simulink model "Model_TranslationEngine64"  (R2022b)
settings: Solver=FixedStepDiscrete  StartTime=0.0  StopTime=5  RelTol=1e-3  EnableMultiTasking=on
InitFcn:
  | % Initialize model
  | ModelSettings=BTConfig.GetModelSettings();
  | 
  | ModelSettings.Validate();
  | 
  | ModelInit;
  | 
  | 
  | % load library data
  | GainLibrary_data;
  | % Load saved values from partition process
  | CapturedConstMask.LoadMapFromFile(bdroot)
StartFcn:
  | % make sure all the simulated RTC requests are found
  | %RTC_SIM_OBJ.ValidateREQs();
undefined symbols (not defined in the file or in its folder): AA, BPLP, Column, NumHFRefBPF, NumHFRefLPF, NumMusicChannels, Row, VolumeMuteConfig
libraries: TuneVar x925, TOP x490, FeaturePath x111, CapturedConstLib x52
(part 24 of 34)

== system Model_TranslationEngine64/ModelPreAmp/DecRate/Medusa5H1/SleepingBeauty/SleepingBeauty/Enabled/SleepingBeautyDR/InnerLink ==
  Captured Tune Const : CapturedConstLib/CapturedConst  TriggerInit=[155 22 255 58]  Role=Automatic
      settings: SourceProductName=Bose Talaria
  FeaturePath : FeaturePath/FeaturePath  FeatureName=SleepingBeautyDR  IsGroup=off  GroupNumber=-1  IsModule=off  TriggerInit=[-415 -561 -300 -454]
      settings: SourceProductName=Bose Talaria
  TOP : TOP/TOP  TriggerInit=[555 -30 785 30]  TopName=ChannelToRamperMap  DataTypeOut=single  BankNumber=0  PreOverlay=false  PostOverlay=false  Role=Automatic
      settings: SourceProductName=Bose Talaria
  TranslateTrigger : TuneVar/TranslateTrigger  TriggerInit=[421 -160 459 -105]
      settings: SourceProductName=Bose Talaria
  TuneTOP : Subsystem  Description=Defines the index at which the index is at the center, i.e. neither towards the left nor the right sides.  mask(Talaria Trivial Tune TOP){TriggerInit=[-595 -93 -425 -37], TopName=Offset, TuneName=Offset, DataTypeOut=single, MaskValue=Config.DefaultOffset, TunabilityNumber=1, MinValue=[], MaxValue=[], BankNumber=0, PreOverlay=false, PostOverlay=false, UseSameName=on}
      mask prompts: TriggerInit "Hidden: MoveFcn redraw"; TopName "Name:"; TuneName "Name of TuneVar:"; DataTypeOut "Data type:"; MaskValue "Default Value:"; TunabilityNumber "Tunability:"; MinValue "Min Value:"; MaxValue "Max Value:"; BankNumber "Target memory bank number:"; PreOverlay "Requires pre-overlay action:"; PostOverlay "Requires post-overlay action:"; UseSameName "Use same name for tune variable and TOP"
      mask help: The TuneTOP block encapsultes a Target Overlay Parameter, a Tune Variable, and a Trivial Translation between them.
      mask init:
      | [ok,activeTopPath,activeTunePath] = TuneTOP_Mask.Init(gcbh);
      settings: MoveFcn=TuneTOP_Mask.CB_TriggerInit(gcbh);
      mask Callback TriggerInit: TuneTOP_Mask.CB_TriggerInit(gcbh);
      mask TypeOptions TopName: TOP/TopName
      mask TypeOptions TuneName: Tune Variable/TuneName
      mask TypeOptions DataTypeOut: TOP/DataTypeOut
      mask TypeOptions MaskValue: Tune Variable/MaskValue
      mask TypeOptions TunabilityNumber: Tune Variable/TunabilityNumber
      mask Callback TunabilityNumber: TuneVarMask.CB_TunabilityNumber(gcbh);
      mask TypeOptions MinValue: Tune Variable/MinValue
      mask TypeOptions MaxValue: Tune Variable/MaxValue
      mask TypeOptions BankNumber: TOP/BankNumber
      mask TypeOptions PreOverlay: TOP/PreOverlay
      mask TypeOptions PostOverlay: TOP/PostOverlay
      mask Callback UseSameName: TuneTOP_Mask.CB_UseSameName(gcbh);
      mask DialogControl toolPanel Prompt: Tuning Tool Hints
      mask DialogControl DescriptionGroup Prompt: Description
      mask DialogControl EditDescription Prompt: Edit Description
      mask DialogControl EditDescription Callback: TuneTOP_Mask.CB_EditDescription(gcbh);
      mask DialogControl TunabilityText Prompt: Easy: Changes nearly every tuning.
      mask DialogControl AdvancedPanel Prompt: Advanced
      mask DialogControl ConvertToFullTranslation Prompt: Irreversible conversion to full translation
      mask DialogControl ConvertToFullTranslation Callback: TuneTOP_Mask.CB_ConvertToFullTranslation(gcbh);
      mask DialogControl ErrorContainer Prompt: Error Messages
      mask Display:
      | % retrieve icon definition
      | [path,w,h] = TuneTOP_Mask.Icon();
      | 
      | % retrieve the block's pixel size
      | pos = get(gcbh,'position');
      | bw = pos(3) - pos(1);
      | bh = pos(4) - pos(2);
      | 
      | % draw centered icon
      | xAdj = bw/2 - w/2 + 5;
      | yAdj = bh/2 - h/2 + 4;
      | for i=1:length(path)
      | 	patch(path(i).x+xAdj, path(i).y+yAdj, path(i).rgb);
      | end
      | 
      | % show the top name or an X
      | if (exist('ok','var') && ok)
      | 	text(bw*0.5, bh*0.2, activeTopPath, 'horizontalAlignment', 'center');
      | 	patch(0,0,[1 1 1]);
      | 	patch(bw,bh,[1 1 1]);
      | else
      | 	tx=bw*0.03;
      | 	ty=bh*0.03;
      | 	patch([0 tx bw bw-tx], [ty 0 bh-ty bh], [1 0 0]);
      | 	patch([0 bw-tx bw tx], [bh-ty 0 ty bh], [1 0 0]);
      | end
  TuneTOP1 : Subsystem  mask(Talaria Trivial Tune TOP){TriggerInit=[135 -393 305 -337], TopName=RampTime, TuneName=RampTime, DataTypeOut=single, MaskValue=30, TunabilityNumber=1, MinValue=[], MaxValue=[], BankNumber=0, PreOverlay=false, PostOverlay=false, UseSameName=on}
      mask prompts: TriggerInit "Hidden: MoveFcn redraw"; TopName "Name:"; TuneName "Name of TuneVar:"; DataTypeOut "Data type:"; MaskValue "Default Value:"; TunabilityNumber "Tunability:"; MinValue "Min Value:"; MaxValue "Max Value:"; BankNumber "Target memory bank number:"; PreOverlay "Requires pre-overlay action:"; PostOverlay "Requires post-overlay action:"; UseSameName "Use same name for tune variable and TOP"
      mask help: The TuneTOP block encapsultes a Target Overlay Parameter, a Tune Variable, and a Trivial Translation between them.
      mask init:
      | [ok,activeTopPath,activeTunePath] = TuneTOP_Mask.Init(gcbh);
      settings: MoveFcn=TuneTOP_Mask.CB_TriggerInit(gcbh);
      mask Callback TriggerInit: TuneTOP_Mask.CB_TriggerInit(gcbh);
      mask TypeOptions TopName: TOP/TopName
      mask TypeOptions TuneName: Tune Variable/TuneName
      mask TypeOptions DataTypeOut: TOP/DataTypeOut
      mask TypeOptions MaskValue: Tune Variable/MaskValue
      mask TypeOptions TunabilityNumber: Tune Variable/TunabilityNumber
      mask Callback TunabilityNumber: TuneVarMask.CB_TunabilityNumber(gcbh);
      mask TypeOptions MinValue: Tune Variable/MinValue
      mask TypeOptions MaxValue: Tune Variable/MaxValue
      mask TypeOptions BankNumber: TOP/BankNumber
      mask TypeOptions PreOverlay: TOP/PreOverlay
      mask TypeOptions PostOverlay: TOP/PostOverlay
      mask Callback UseSameName: TuneTOP_Mask.CB_UseSameName(gcbh);
      mask DialogControl toolPanel Prompt: Tuning Tool Hints
      mask DialogControl DescriptionGroup Prompt: Description
      mask DialogControl EditDescription Prompt: Edit Description
      mask DialogControl EditDescription Callback: TuneTOP_Mask.CB_EditDescription(gcbh);
      mask DialogControl TunabilityText Prompt: Easy: Changes nearly every tuning.
      mask DialogControl AdvancedPanel Prompt: Advanced
      mask DialogControl ConvertToFullTranslation Prompt: Irreversible conversion to full translation
      mask DialogControl ConvertToFullTranslation Callback: TuneTOP_Mask.CB_ConvertToFullTranslation(gcbh);
      mask DialogControl ErrorContainer Prompt: Error Messages
      mask Display:
      | % retrieve icon definition
      | [path,w,h] = TuneTOP_Mask.Icon();
      | 
      | % retrieve the block's pixel size
      | pos = get(gcbh,'position');
      | bw = pos(3) - pos(1);
      | bh = pos(4) - pos(2);
      | 
      | % draw centered icon
      | xAdj = bw/2 - w/2 + 5;
      | yAdj = bh/2 - h/2 + 4;
      | for i=1:length(path)
      | 	patch(path(i).x+xAdj, path(i).y+yAdj, path(i).rgb);
      | end
      | 
      | % show the top name or an X
      | if (exist('ok','var') && ok)
      | 	text(bw*0.5, bh*0.2, activeTopPath, 'horizontalAlignment', 'center');
      | 	patch(0,0,[1 1 1]);
      | 	patch(bw,bh,[1 1 1]);
      | else
      | 	tx=bw*0.03;
      | 	ty=bh*0.03;
      | 	patch([0 tx bw bw-tx], [ty 0 bh-ty bh], [1 0 0]);
      | 	patch([0 bw-tx bw tx], [bh-ty 0 ty bh], [1 0 0]);
      | end
  TuneTOP2 : Subsystem  Description=Defines the index at which the index is at the center, i.e. neither towards the left nor the right sides.  mask(Talaria Trivial Tune TOP){TriggerInit=[-595 17 -425 73], TopName=MutesBass, TuneName=MutesBass, DataTypeOut=single, MaskValue=Config.DefaultSilentExtremeMutesBass, TunabilityNumber=1, MinValue=[], MaxValue=[], BankNumber=0, PreOverlay=false, PostOverlay=false, UseSameName=on}
      mask prompts: TriggerInit "Hidden: MoveFcn redraw"; TopName "Name:"; TuneName "Name of TuneVar:"; DataTypeOut "Data type:"; MaskValue "Default Value:"; TunabilityNumber "Tunability:"; MinValue "Min Value:"; MaxValue "Max Value:"; BankNumber "Target memory bank number:"; PreOverlay "Requires pre-overlay action:"; PostOverlay "Requires post-overlay action:"; UseSameName "Use same name for tune variable and TOP"
      mask help: The TuneTOP block encapsultes a Target Overlay Parameter, a Tune Variable, and a Trivial Translation between them.
      mask init:
      | [ok,activeTopPath,activeTunePath] = TuneTOP_Mask.Init(gcbh);
      settings: MoveFcn=TuneTOP_Mask.CB_TriggerInit(gcbh);
      mask Callback TriggerInit: TuneTOP_Mask.CB_TriggerInit(gcbh);
      mask TypeOptions TopName: TOP/TopName
      mask TypeOptions TuneName: Tune Variable/TuneName
      mask TypeOptions DataTypeOut: TOP/DataTypeOut
      mask TypeOptions MaskValue: Tune Variable/MaskValue
      mask TypeOptions TunabilityNumber: Tune Variable/TunabilityNumber
      mask Callback TunabilityNumber: TuneVarMask.CB_TunabilityNumber(gcbh);
      mask TypeOptions MinValue: Tune Variable/MinValue
      mask TypeOptions MaxValue: Tune Variable/MaxValue
      mask TypeOptions BankNumber: TOP/BankNumber
      mask TypeOptions PreOverlay: TOP/PreOverlay
      mask TypeOptions PostOverlay: TOP/PostOverlay
      mask Callback UseSameName: TuneTOP_Mask.CB_UseSameName(gcbh);
      mask DialogControl toolPanel Prompt: Tuning Tool Hints
      mask DialogControl DescriptionGroup Prompt: Description
      mask DialogControl EditDescription Prompt: Edit Description
      mask DialogControl EditDescription Callback: TuneTOP_Mask.CB_EditDescription(gcbh);
      mask DialogControl TunabilityText Prompt: Easy: Changes nearly every tuning.
      mask DialogControl AdvancedPanel Prompt: Advanced
      mask DialogControl ConvertToFullTranslation Prompt: Irreversible conversion to full translation
      mask DialogControl ConvertToFullTranslation Callback: TuneTOP_Mask.CB_ConvertToFullTranslation(gcbh);
      mask DialogControl ErrorContainer Prompt: Error Messages
      mask Display:
      | % retrieve icon definition
      | [path,w,h] = TuneTOP_Mask.Icon();
      | 
      | % retrieve the block's pixel size
      | pos = get(gcbh,'position');
      | bw = pos(3) - pos(1);
      | bh = pos(4) - pos(2);
      | 
      | % draw centered icon
      | xAdj = bw/2 - w/2 + 5;
      | yAdj = bh/2 - h/2 + 4;
      | for i=1:length(path)
      | 	patch(path(i).x+xAdj, path(i).y+yAdj, path(i).rgb);
      | end
      | 
      | % show the top name or an X
      | if (exist('ok','var') && ok)
      | 	text(bw*0.5, bh*0.2, activeTopPath, 'horizontalAlignment', 'center');
      | 	patch(0,0,[1 1 1]);
      | 	patch(bw,bh,[1 1 1]);
      | else
      | 	tx=bw*0.03;
      | 	ty=bh*0.03;
      | 	patch([0 tx bw bw-tx], [ty 0 bh-ty bh], [1 0 0]);
      | 	patch([0 bw-tx bw tx], [bh-ty 0 ty bh], [1 0 0]);
      | end
  TuneVarChannelRamperMap : TuneVar/TuneVar  TuneName=ChannelToRamperMap  SpecifyMaxSize=off  VariableDim=1 (Row)  MaxSize=[1 1]  TunabilityNumber=1  MinValue=[]  MaxValue=[]  TriggerInit=[70 -65 280 -15]  MaskValue=Config.ChanToRampMap
      settings: SourceProductName=Bose Talaria
  TuneVarTable : Subsystem
  channel_ramper_translation : MATLAB Function  TreatAsAtomicUnit=on  mask{MaskNumRampers=Config.NumRampers}
  wires:
  TranslateTrigger/1 -> channel_ramper_translation/Trigger
  TuneVarChannelRamperMap/1 -> channel_ramper_translation/1(TuneChanRampMap)  "ChannelToRamperMap"
  channel_ramper_translation/1(ChanRampMap) -> TOP/1
  Captured Tune Const/1 -> channel_ramper_translation/2(channelCount)

== system Model_TranslationEngine64/ModelPreAmp/DecRate/Medusa5H1/SleepingBeauty/SleepingBeauty/Enabled/SleepingBeautyFR/InnerLink ==
  Captured Tune Const : CapturedConstLib/CapturedConst  TriggerInit=[155 22 255 58]  Role=Automatic
      settings: SourceProductName=Bose Talaria
  FeaturePath : FeaturePath/FeaturePath  FeatureName=SleepingBeautyFR  IsGroup=off  GroupNumber=-1  IsModule=off  TriggerInit=[-415 -561 -300 -454]
      settings: SourceProductName=Bose Talaria
  TOP : TOP/TOP  TriggerInit=[555 -30 785 30]  TopName=ChannelToRamperMap  DataTypeOut=single  BankNumber=0  PreOverlay=false  PostOverlay=false  Role=Automatic
      settings: SourceProductName=Bose Talaria
  TranslateTrigger : TuneVar/TranslateTrigger  TriggerInit=[421 -160 459 -105]
      settings: SourceProductName=Bose Talaria
  TuneTOP : Subsystem  Description=Defines the index at which the index is at the center, i.e. neither towards the left nor the right sides.  mask(Talaria Trivial Tune TOP){TriggerInit=[-595 -93 -425 -37], TopName=Offset, TuneName=Offset, DataTypeOut=single, MaskValue=Config.DefaultOffset, TunabilityNumber=1, MinValue=[], MaxValue=[], BankNumber=0, PreOverlay=false, PostOverlay=false, UseSameName=on}
      mask prompts: TriggerInit "Hidden: MoveFcn redraw"; TopName "Name:"; TuneName "Name of TuneVar:"; DataTypeOut "Data type:"; MaskValue "Default Value:"; TunabilityNumber "Tunability:"; MinValue "Min Value:"; MaxValue "Max Value:"; BankNumber "Target memory bank number:"; PreOverlay "Requires pre-overlay action:"; PostOverlay "Requires post-overlay action:"; UseSameName "Use same name for tune variable and TOP"
      mask help: The TuneTOP block encapsultes a Target Overlay Parameter, a Tune Variable, and a Trivial Translation between them.
      mask init:
      | [ok,activeTopPath,activeTunePath] = TuneTOP_Mask.Init(gcbh);
      settings: MoveFcn=TuneTOP_Mask.CB_TriggerInit(gcbh);
      mask Callback TriggerInit: TuneTOP_Mask.CB_TriggerInit(gcbh);
      mask TypeOptions TopName: TOP/TopName
      mask TypeOptions TuneName: Tune Variable/TuneName
      mask TypeOptions DataTypeOut: TOP/DataTypeOut
      mask TypeOptions MaskValue: Tune Variable/MaskValue
      mask TypeOptions TunabilityNumber: Tune Variable/TunabilityNumber
      mask Callback TunabilityNumber: TuneVarMask.CB_TunabilityNumber(gcbh);
      mask TypeOptions MinValue: Tune Variable/MinValue
      mask TypeOptions MaxValue: Tune Variable/MaxValue
      mask TypeOptions BankNumber: TOP/BankNumber
      mask TypeOptions PreOverlay: TOP/PreOverlay
      mask TypeOptions PostOverlay: TOP/PostOverlay
      mask Callback UseSameName: TuneTOP_Mask.CB_UseSameName(gcbh);
      mask DialogControl toolPanel Prompt: Tuning Tool Hints
      mask DialogControl DescriptionGroup Prompt: Description
      mask DialogControl EditDescription Prompt: Edit Description
      mask DialogControl EditDescription Callback: TuneTOP_Mask.CB_EditDescription(gcbh);
      mask DialogControl TunabilityText Prompt: Easy: Changes nearly every tuning.
      mask DialogControl AdvancedPanel Prompt: Advanced
      mask DialogControl ConvertToFullTranslation Prompt: Irreversible conversion to full translation
      mask DialogControl ConvertToFullTranslation Callback: TuneTOP_Mask.CB_ConvertToFullTranslation(gcbh);
      mask DialogControl ErrorContainer Prompt: Error Messages
      mask Display:
      | % retrieve icon definition
      | [path,w,h] = TuneTOP_Mask.Icon();
      | 
      | % retrieve the block's pixel size
      | pos = get(gcbh,'position');
      | bw = pos(3) - pos(1);
      | bh = pos(4) - pos(2);
      | 
      | % draw centered icon
      | xAdj = bw/2 - w/2 + 5;
      | yAdj = bh/2 - h/2 + 4;
      | for i=1:length(path)
      | 	patch(path(i).x+xAdj, path(i).y+yAdj, path(i).rgb);
      | end
      | 
      | % show the top name or an X
      | if (exist('ok','var') && ok)
      | 	text(bw*0.5, bh*0.2, activeTopPath, 'horizontalAlignment', 'center');
      | 	patch(0,0,[1 1 1]);
      | 	patch(bw,bh,[1 1 1]);
      | else
      | 	tx=bw*0.03;
      | 	ty=bh*0.03;
      | 	patch([0 tx bw bw-tx], [ty 0 bh-ty bh], [1 0 0]);
      | 	patch([0 bw-tx bw tx], [bh-ty 0 ty bh], [1 0 0]);
      | end
  TuneTOP1 : Subsystem  mask(Talaria Trivial Tune TOP){TriggerInit=[135 -393 305 -337], TopName=RampTime, TuneName=RampTime, DataTypeOut=single, MaskValue=30, TunabilityNumber=1, MinValue=[], MaxValue=[], BankNumber=0, PreOverlay=false, PostOverlay=false, UseSameName=on}
      mask prompts: TriggerInit "Hidden: MoveFcn redraw"; TopName "Name:"; TuneName "Name of TuneVar:"; DataTypeOut "Data type:"; MaskValue "Default Value:"; TunabilityNumber "Tunability:"; MinValue "Min Value:"; MaxValue "Max Value:"; BankNumber "Target memory bank number:"; PreOverlay "Requires pre-overlay action:"; PostOverlay "Requires post-overlay action:"; UseSameName "Use same name for tune variable and TOP"
      mask help: The TuneTOP block encapsultes a Target Overlay Parameter, a Tune Variable, and a Trivial Translation between them.
      mask init:
      | [ok,activeTopPath,activeTunePath] = TuneTOP_Mask.Init(gcbh);
      settings: MoveFcn=TuneTOP_Mask.CB_TriggerInit(gcbh);
      mask Callback TriggerInit: TuneTOP_Mask.CB_TriggerInit(gcbh);
      mask TypeOptions TopName: TOP/TopName
      mask TypeOptions TuneName: Tune Variable/TuneName
      mask TypeOptions DataTypeOut: TOP/DataTypeOut
      mask TypeOptions MaskValue: Tune Variable/MaskValue
      mask TypeOptions TunabilityNumber: Tune Variable/TunabilityNumber
      mask Callback TunabilityNumber: TuneVarMask.CB_TunabilityNumber(gcbh);
      mask TypeOptions MinValue: Tune Variable/MinValue
      mask TypeOptions MaxValue: Tune Variable/MaxValue
      mask TypeOptions BankNumber: TOP/BankNumber
      mask TypeOptions PreOverlay: TOP/PreOverlay
      mask TypeOptions PostOverlay: TOP/PostOverlay
      mask Callback UseSameName: TuneTOP_Mask.CB_UseSameName(gcbh);
      mask DialogControl toolPanel Prompt: Tuning Tool Hints
      mask DialogControl DescriptionGroup Prompt: Description
      mask DialogControl EditDescription Prompt: Edit Description
      mask DialogControl EditDescription Callback: TuneTOP_Mask.CB_EditDescription(gcbh);
      mask DialogControl TunabilityText Prompt: Easy: Changes nearly every tuning.
      mask DialogControl AdvancedPanel Prompt: Advanced
      mask DialogControl ConvertToFullTranslation Prompt: Irreversible conversion to full translation
      mask DialogControl ConvertToFullTranslation Callback: TuneTOP_Mask.CB_ConvertToFullTranslation(gcbh);
      mask DialogControl ErrorContainer Prompt: Error Messages
      mask Display:
      | % retrieve icon definition
      | [path,w,h] = TuneTOP_Mask.Icon();
      | 
      | % retrieve the block's pixel size
      | pos = get(gcbh,'position');
      | bw = pos(3) - pos(1);
      | bh = pos(4) - pos(2);
      | 
      | % draw centered icon
      | xAdj = bw/2 - w/2 + 5;
      | yAdj = bh/2 - h/2 + 4;
      | for i=1:length(path)
      | 	patch(path(i).x+xAdj, path(i).y+yAdj, path(i).rgb);
      | end
      | 
      | % show the top name or an X
      | if (exist('ok','var') && ok)
      | 	text(bw*0.5, bh*0.2, activeTopPath, 'horizontalAlignment', 'center');
      | 	patch(0,0,[1 1 1]);
      | 	patch(bw,bh,[1 1 1]);
      | else
      | 	tx=bw*0.03;
      | 	ty=bh*0.03;
      | 	patch([0 tx bw bw-tx], [ty 0 bh-ty bh], [1 0 0]);
      | 	patch([0 bw-tx bw tx], [bh-ty 0 ty bh], [1 0 0]);
      | end
  TuneTOP2 : Subsystem  Description=Defines the index at which the index is at the center, i.e. neither towards the left nor the right sides.  mask(Talaria Trivial Tune TOP){TriggerInit=[-595 17 -425 73], TopName=MutesBass, TuneName=MutesBass, DataTypeOut=single, MaskValue=Config.DefaultSilentExtremeMutesBass, TunabilityNumber=1, MinValue=[], MaxValue=[], BankNumber=0, PreOverlay=false, PostOverlay=false, UseSameName=on}
      mask prompts: TriggerInit "Hidden: MoveFcn redraw"; TopName "Name:"; TuneName "Name of TuneVar:"; DataTypeOut "Data type:"; MaskValue "Default Value:"; TunabilityNumber "Tunability:"; MinValue "Min Value:"; MaxValue "Max Value:"; BankNumber "Target memory bank number:"; PreOverlay "Requires pre-overlay action:"; PostOverlay "Requires post-overlay action:"; UseSameName "Use same name for tune variable and TOP"
      mask help: The TuneTOP block encapsultes a Target Overlay Parameter, a Tune Variable, and a Trivial Translation between them.
      mask init:
      | [ok,activeTopPath,activeTunePath] = TuneTOP_Mask.Init(gcbh);
      settings: MoveFcn=TuneTOP_Mask.CB_TriggerInit(gcbh);
      mask Callback TriggerInit: TuneTOP_Mask.CB_TriggerInit(gcbh);
      mask TypeOptions TopName: TOP/TopName
      mask TypeOptions TuneName: Tune Variable/TuneName
      mask TypeOptions DataTypeOut: TOP/DataTypeOut
      mask TypeOptions MaskValue: Tune Variable/MaskValue
      mask TypeOptions TunabilityNumber: Tune Variable/TunabilityNumber
      mask Callback TunabilityNumber: TuneVarMask.CB_TunabilityNumber(gcbh);
      mask TypeOptions MinValue: Tune Variable/MinValue
      mask TypeOptions MaxValue: Tune Variable/MaxValue
      mask TypeOptions BankNumber: TOP/BankNumber
      mask TypeOptions PreOverlay: TOP/PreOverlay
      mask TypeOptions PostOverlay: TOP/PostOverlay
      mask Callback UseSameName: TuneTOP_Mask.CB_UseSameName(gcbh);
      mask DialogControl toolPanel Prompt: Tuning Tool Hints
      mask DialogControl DescriptionGroup Prompt: Description
      mask DialogControl EditDescription Prompt: Edit Description
      mask DialogControl EditDescription Callback: TuneTOP_Mask.CB_EditDescription(gcbh);
      mask DialogControl TunabilityText Prompt: Easy: Changes nearly every tuning.
      mask DialogControl AdvancedPanel Prompt: Advanced
      mask DialogControl ConvertToFullTranslation Prompt: Irreversible conversion to full translation
      mask DialogControl ConvertToFullTranslation Callback: TuneTOP_Mask.CB_ConvertToFullTranslation(gcbh);
      mask DialogControl ErrorContainer Prompt: Error Messages
      mask Display:
      | % retrieve icon definition
      | [path,w,h] = TuneTOP_Mask.Icon();
      | 
      | % retrieve the block's pixel size
      | pos = get(gcbh,'position');
      | bw = pos(3) - pos(1);
      | bh = pos(4) - pos(2);
      | 
      | % draw centered icon
      | xAdj = bw/2 - w/2 + 5;
      | yAdj = bh/2 - h/2 + 4;
      | for i=1:length(path)
      | 	patch(path(i).x+xAdj, path(i).y+yAdj, path(i).rgb);
      | end
      | 
      | % show the top name or an X
      | if (exist('ok','var') && ok)
      | 	text(bw*0.5, bh*0.2, activeTopPath, 'horizontalAlignment', 'center');
      | 	patch(0,0,[1 1 1]);
      | 	patch(bw,bh,[1 1 1]);
      | else
      | 	tx=bw*0.03;
      | 	ty=bh*0.03;
      | 	patch([0 tx bw bw-tx], [ty 0 bh-ty bh], [1 0 0]);
      | 	patch([0 bw-tx bw tx], [bh-ty 0 ty bh], [1 0 0]);
      | end
  TuneVarChannelRamperMap : TuneVar/TuneVar  TuneName=ChannelToRamperMap  SpecifyMaxSize=off  VariableDim=1 (Row)  MaxSize=[1 1]  TunabilityNumber=1  MinValue=[]  MaxValue=[]  TriggerInit=[70 -65 280 -15]  MaskValue=Config.ChanToRampMap
      settings: SourceProductName=Bose Talaria
  TuneVarTable : Subsystem
  channel_ramper_translation : MATLAB Function  TreatAsAtomicUnit=on  mask{MaskNumRampers=Config.NumRampers}
  wires:
  TranslateTrigger/1 -> channel_ramper_translation/Trigger
  TuneVarChannelRamperMap/1 -> channel_ramper_translation/1(TuneChanRampMap)  "ChannelToRamperMap"
  channel_ramper_translation/1(ChanRampMap) -> TOP/1
  Captured Tune Const/1 -> channel_ramper_translation/2(channelCount)

== system Model_TranslationEngine64/ModelPreAmp/DecRate/Medusa5H1/VLS/Crosstalk Cancellation/Pooliir with Non-Trivial Translations/InnerLink/PoolIirTunableWithReset ==
  CapturedTuneConst : CapturedConstLib/CapturedConst  TriggerInit=[-600 302 -500 338]  Role=Automatic
      settings: SourceProductName=Bose Talaria
  FeaturePath : FeaturePath/FeaturePath  FeatureName=IIR  IsGroup=off  GroupNumber=-1  IsModule=off  TriggerInit=[-750 -81 -635 26]
      settings: SourceProductName=Bose Talaria
  TOP : TOP/TOP  TriggerInit=[-145 187 5 243]  TopName=PooliirNumStages  DataTypeOut=uint32  BankNumber=0  PreOverlay=false  PostOverlay=Config.VariantObj.PostOverlayRequired  Role=Automatic
      settings: SourceProductName=Bose Talaria
  TOP1 : TOP/TOP  TriggerInit=[-140 277 10 333]  TopName=pooliirCoeffs  DataTypeOut=single  BankNumber=0  PreOverlay=false  PostOverlay=Config.VariantObj.PostOverlayRequired  Role=Automatic
      settings: SourceProductName=Bose Talaria
  TranslateTrigger : TuneVar/TranslateTrigger  TriggerInit=[-339 35 -301 90]
      settings: SourceProductName=Bose Talaria
  Translation : MATLAB Function  TreatAsAtomicUnit=on  mask{MaxNumStages=Config.MaxNumStages, VariantUint8=Config.Variant.Uint8Str}
      mask prompts: VariantUint8 "Variant"
  Tune Variable1 : TuneVar/TuneVar  TuneName=numStages  SpecifyMaxSize=off  VariableDim=1 (Row)  MaxSize=[1 1]  TunabilityNumber=1  MinValue=[]  MaxValue=[]  TriggerInit=[-750 235 -580 285]  MaskValue=Config.TuneDefaults.NumStages
      settings: SourceProductName=Bose Talaria
  Tune Variable2 : TuneVar/TuneVar  TuneName=sosCoefficients  SpecifyMaxSize=on  VariableDim=1 (Row)  MaxSize=[Config.MaxNumStages 6]  TunabilityNumber=1  MinValue=[]  MaxValue=[]  TriggerInit=[-750 175 -580 225]  MaskValue=Config.TuneDefaults.SosCoefficients
      settings: SourceProductName=Bose Talaria
  wires:
  CapturedTuneConst/1 -> Translation/3(NumChannels)
  Tune Variable1/1 -> Translation/2(NumStages)  "numStages"
  Translation/1(PoolNumStages) -> TOP/1
  Translation/2(PoolCoeffs) -> TOP1/1
  Tune Variable2/1 -> Translation/1(RawSOS)  "sosCoefficients"
  TranslateTrigger/1 -> Translation/Trigger

== system Model_TranslationEngine64/ModelPreAmp/PreAmpPart1/NEARPreAmp/Monoizer/Monoizer/MonoizerStereo/MonoizerCalc/TuneTOP1 ==
  TOP : TOP/TOP  TriggerInit=[440 20 585 80]  TopName=G  DataTypeOut=single  BankNumber=BankNumber  PreOverlay=PreOverlay  PostOverlay=PostOverlay  Role=Automatic
      settings: SourceProductName=Bose Talaria
  TrivialTranslation : TuneVar/TrivialTranslation  TriggerInit=[300 28 350 72]
      settings: SourceProductName=Bose Talaria
  Tune Variable : TuneVar/TuneVar  TuneName=G  SpecifyMaxSize=off  VariableDim=1 (Row)  MaxSize=[1 1]  TunabilityNumber=1  MinValue=MinValue  MaxValue=MaxValue  TriggerInit=[20 25 190 75]  MaskValue=MaskValue
      settings: SourceProductName=Bose Talaria
  wires:
  Tune Variable/1 -> TrivialTranslation/1  "G"
  TrivialTranslation/1 -> TOP/1

== system Model_TranslationEngine64/ModelPreAmp/DecRate/AudioPilot35/Audiopilot_3_5/NoiseEstimationVariant/RegularNoiseEstimation/HFNoiseEstimatorCoh/HfNoiseMusicSeparation /RefPowerMin ==
  RefPowerMin : TOP/TOP  TriggerInit=[440 20 585 80]  TopName=RefPowerMin  DataTypeOut=single  BankNumber=0  PreOverlay=false  PostOverlay=false  Role=Automatic
      settings: SourceProductName=Bose Talaria
  TranslateTrigger : TuneVar/TranslateTrigger  TriggerInit=[306 -100 344 -45]
      settings: SourceProductName=Bose Talaria
  Tune Variable : TuneVar/TuneVar  TuneName=RefPowerMinDb  SpecifyMaxSize=off  VariableDim=1 (Row)  MaxSize=[1 1]  TunabilityNumber=1  MinValue=[]  MaxValue=[]  TriggerInit=[-25 25 145 75]  MaskValue=Config.RefPowerMinDb
      settings: SourceProductName=Bose Talaria
  undB : MATLAB Function  TreatAsAtomicUnit=on
  wires:
  Tune Variable/1 -> undB/1(Tune)  "RefPowerMinDb"
  undB/1(TOP) -> RefPowerMin/1
  TranslateTrigger/1 -> undB/Trigger

== system Model_TranslationEngine64/ModelPreAmp/DecRate/AudioPilot35/Audiopilot_3_5/NoiseEstimationVariant/RegularNoiseEstimation/HFNoiseEstimatorCoh/PostProcessing/HfImpulseRejection ==
  note: Impulse and Speech Rejection
  ComputeSmoothingFactor : Subsystem
  FeaturePath : FeaturePath/FeaturePath  FeatureName=ImpulseRejection  IsGroup=off  GroupNumber=-1  IsModule=off  TriggerInit=[750 304 1100 406]
      settings: SourceProductName=Bose Talaria
  "IntermediateCalculation1 " : Subsystem
  MinSearch : Subsystem
  SmoothingNoiseFloor : Subsystem

== system Model_TranslationEngine64/ModelPreAmp/DecRate/AudioPilot35/Audiopilot_3_5/NoiseEstimationVariant/RegularNoiseEstimation/HFNoiseEstimatorCoh/PostProcessing/HfSlew ==
  note: Slew for High-Frequency Noise Esimate
  FeaturePath : FeaturePath/FeaturePath  FeatureName=Slew  IsGroup=off  GroupNumber=-1  IsModule=off  TriggerInit=[85 39 200 146]
      settings: SourceProductName=Bose Talaria
  attack : Subsystem
  decay : Subsystem
  threshold : Subsystem  mask(Talaria Trivial Tune TOP){TriggerInit=[30 282 255 318], TopName=ThresholdDb, TuneName=ThresholdDb, DataTypeOut=single, MaskValue=Config.SlewThresholdDb, TunabilityNumber=1, MinValue=[], MaxValue=[], BankNumber=0, PreOverlay=false, PostOverlay=false, UseSameName=on}
      mask prompts: TriggerInit "Hidden: MoveFcn redraw"; TopName "Name:"; TuneName "Name of TuneVar:"; DataTypeOut "Data type:"; MaskValue "Default Value:"; TunabilityNumber "Tunability:"; MinValue "Min Value:"; MaxValue "Max Value:"; BankNumber "Target memory bank number:"; PreOverlay "Requires pre-overlay action:"; PostOverlay "Requires post-overlay action:"; UseSameName "Use same name for tune variable and TOP"
      mask help: The TuneTOP block encapsultes a Target Overlay Parameter, a Tune Variable, and a Trivial Translation between them.
      mask init:
      | [ok,activeTopPath,activeTunePath] = TuneTOP_Mask.Init(gcbh);
      settings: MoveFcn=TuneTOP_Mask.CB_TriggerInit(gcbh);
      mask Callback TriggerInit: TuneTOP_Mask.CB_TriggerInit(gcbh);
      mask TypeOptions TopName: TOP/TopName
      mask TypeOptions TuneName: Tune Variable/TuneName
      mask TypeOptions DataTypeOut: TOP/DataTypeOut
      mask TypeOptions MaskValue: Tune Variable/MaskValue
      mask TypeOptions TunabilityNumber: Tune Variable/TunabilityNumber
      mask Callback TunabilityNumber: TuneVarMask.CB_TunabilityNumber(gcbh);
      mask TypeOptions MinValue: Tune Variable/MinValue
      mask TypeOptions MaxValue: Tune Variable/MaxValue
      mask TypeOptions BankNumber: TOP/BankNumber
      mask TypeOptions PreOverlay: TOP/PreOverlay
      mask TypeOptions PostOverlay: TOP/PostOverlay
      mask Callback UseSameName: TuneTOP_Mask.CB_UseSameName(gcbh);
      mask DialogControl toolPanel Prompt: Tuning Tool Hints
      mask DialogControl DescriptionGroup Prompt: Description
      mask DialogControl EditDescription Prompt: Edit Description
      mask DialogControl EditDescription Callback: TuneTOP_Mask.CB_EditDescription(gcbh);
      mask DialogControl TunabilityText Prompt: Easy: Changes nearly every tuning.
      mask DialogControl AdvancedPanel Prompt: Advanced
      mask DialogControl ConvertToFullTranslation Prompt: Irreversible conversion to full translation
      mask DialogControl ConvertToFullTranslation Callback: TuneTOP_Mask.CB_ConvertToFullTranslation(gcbh);
      mask DialogControl ErrorContainer Prompt: Error Messages
      mask Display:
      | % retrieve icon definition
      | [path,w,h] = TuneTOP_Mask.Icon();
      | 
      | % retrieve the block's pixel size
      | pos = get(gcbh,'position');
      | bw = pos(3) - pos(1);
      | bh = pos(4) - pos(2);
      | 
      | % draw centered icon
      | xAdj = bw/2 - w/2 + 5;
      | yAdj = bh/2 - h/2 + 4;
      | for i=1:length(path)
      | 	patch(path(i).x+xAdj, path(i).y+yAdj, path(i).rgb);
      | end
      | 
      | % show the top name or an X
      | if (exist('ok','var') && ok)
      | 	text(bw*0.5, bh*0.2, activeTopPath, 'horizontalAlignment', 'center');
      | 	patch(0,0,[1 1 1]);
      | 	patch(bw,bh,[1 1 1]);
      | else
      | 	tx=bw*0.03;
      | 	ty=bh*0.03;
      | 	patch([0 tx bw bw-tx], [ty 0 bh-ty bh], [1 0 0]);
      | 	patch([0 bw-tx bw tx], [bh-ty 0 ty bh], [1 0 0]);
      | end

== system Model_TranslationEngine64/ModelPreAmp/DecRate/AudioPilot35/Audiopilot_3_5/NoiseEstimationVariant/RegularNoiseEstimation/HFNoiseEstimatorCoh/PostProcessing/offset ==
  TOP : TOP/TOP  TriggerInit=[440 20 585 80]  TopName=OffsetDb  DataTypeOut=single  BankNumber=BankNumber  PreOverlay=PreOverlay  PostOverlay=PostOverlay  Role=Automatic
      settings: SourceProductName=Bose Talaria
  TrivialTranslation : TuneVar/TrivialTranslation  TriggerInit=[300 28 350 72]
      settings: SourceProductName=Bose Talaria
  Tune Variable : TuneVar/TuneVar  TuneName=OffsetDb  SpecifyMaxSize=off  VariableDim=1 (Row)  MaxSize=[1 1]  TunabilityNumber=1  MinValue=MinValue  MaxValue=MaxValue  TriggerInit=[20 25 190 75]  MaskValue=MaskValue
      settings: SourceProductName=Bose Talaria
  wires:
  TrivialTranslation/1 -> TOP/1
  Tune Variable/1 -> TrivialTranslation/1  "OffsetDb"

== system Model_TranslationEngine64/ModelPreAmp/DecRate/AudioPilot35/Audiopilot_3_5/NoiseEstimationVariant/RegularNoiseEstimation/HFNoiseEstimatorCoh/PreProcessing/Anti-Aliasing Filter ==
  InnerLink : Subsystem  mask(Bose Pool IIR Tunable){FeatureName=PreprocessAntiAlias, Config=InnerLinkConfig}
      mask prompts: FeatureName "Filter name/purpose"; Config "PoolIirTunableConfig"
      mask help:
      | Pool IIR Tunable is a configurable multi-channel IIR filter that supports one or more channels. This block offers flexibility of tuning the number of stages and coefficients. Different filter coefficients and number of stages (biquads) can be used for each channel filter. The Pool IIR Tunable block supports different implementations, which could be configured at build-time:
      |
      | (i)   Generic: IIR filter code not optimized for any processor
      | (ii)  SharcCore: IIR filters executing on core (uses pooliir.asm CRL)
      | (iii) SharcGulAccel: IIR filters executing on IIR hardware accelerator, offloading MIPS usage from core
      | (iv) SharcGxpAccel: IIR filters take advantage of additional accelerators available on GXP processor
      | (v)  Hexagon: TBD
      |
      | NOTE: When using Pool IIR for Sharc-plus based processors, the codeWorkMemory buffer and input buffer should always be mapped to L1 memory to optimize MIPS utilization and avoid audio artifacts.
      |
      | For more information, please see 'Help'.
      mask init:
      | blkh=gcbh;
      | Config=BTConfig.Assert(blkh,Config);
      | 
      | Config.Validate();
      | Config.DoMaskInit(blkh);
      mask Help:
      | <b>Input signals: </b>
      | AudioIn: input channels [frame size x number of channels]
      | 
      | <b>Output signals: </b>
      | AudioOut: output channels [frame size x number of channels]
      | 
      | <b>Mask parameters: </b>
      | PoolIirTunableConfig
      | Filter name/purpose
      mask TypeOptions FeatureName: PoolIirTunableWithReset/FeatureName
      mask Display: DrawPoolIirIcon;

== system Model_TranslationEngine64/ModelPreAmp/DecRate/AudioPilot35/Audiopilot_3_5/NoiseEstimationVariant/RegularNoiseEstimation/HFNoiseEstimatorCoh/PreProcessing/Bandpass or Lowpass Filter ==
  InnerLink : Subsystem  mask(Bose Pool IIR Tunable){FeatureName=PreprocessBandpassLowpass, Config=InnerLinkConfig}
      mask prompts: FeatureName "Filter name/purpose"; Config "PoolIirTunableConfig"
      mask help:
      | Pool IIR Tunable is a configurable multi-channel IIR filter that supports one or more channels. This block offers flexibility of tuning the number of stages and coefficients. Different filter coefficients and number of stages (biquads) can be used for each channel filter. The Pool IIR Tunable block supports different implementations, which could be configured at build-time:
      |
      | (i)   Generic: IIR filter code not optimized for any processor
      | (ii)  SharcCore: IIR filters executing on core (uses pooliir.asm CRL)
      | (iii) SharcGulAccel: IIR filters executing on IIR hardware accelerator, offloading MIPS usage from core
      | (iv) SharcGxpAccel: IIR filters take advantage of additional accelerators available on GXP processor
      | (v)  Hexagon: TBD
      |
      | NOTE: When using Pool IIR for Sharc-plus based processors, the codeWorkMemory buffer and input buffer should always be mapped to L1 memory to optimize MIPS utilization and avoid audio artifacts.
      |
      | For more information, please see 'Help'.
      mask init:
      | blkh=gcbh;
      | Config=BTConfig.Assert(blkh,Config);
      | 
      | Config.Validate();
      | Config.DoMaskInit(blkh);
      mask Help:
      | <b>Input signals: </b>
      | AudioIn: input channels [frame size x number of channels]
      | 
      | <b>Output signals: </b>
      | AudioOut: output channels [frame size x number of channels]
      | 
      | <b>Mask parameters: </b>
      | PoolIirTunableConfig
      | Filter name/purpose
      mask TypeOptions FeatureName: PoolIirTunableWithReset/FeatureName
      mask Display: DrawPoolIirIcon;

== system Model_TranslationEngine64/ModelPreAmp/DecRate/AudioPilot35/Audiopilot_3_5/NoiseEstimationVariant/RegularNoiseEstimation/HFNoiseEstimatorCoh/ReferenceLatency/RefLatency ==
  Captured Tune Const : CapturedConstLib/CapturedConst  TriggerInit=[-195 162 -95 198]  Role=Automatic
      settings: SourceProductName=Bose Talaria
  TOP : TOP/TOP  TriggerInit=[85 129 255 171]  TopName=RefLatencySamples  DataTypeOut=int32  BankNumber=0  PreOverlay=false  PostOverlay=false  Role=Automatic
      settings: SourceProductName=Bose Talaria
  TranslateTrigger : TuneVar/TranslateTrigger  TriggerInit=[-24 -20 14 35]
      settings: SourceProductName=Bose Talaria
  Tune Variable : TuneVar/TuneVar  TuneName=RefLatencyMs  SpecifyMaxSize=off  VariableDim=1 (Row)  MaxSize=[1 1]  TunabilityNumber=1  MinValue=[]  MaxValue=[]  TriggerInit=[-435 90 -240 140]  MaskValue=Config.RefLatencyMsec
      settings: SourceProductName=Bose Talaria
  ms2samples : MATLAB Function  TreatAsAtomicUnit=on
  wires:
  TranslateTrigger/1 -> ms2samples/Trigger
  Tune Variable/1 -> ms2samples/1(DelayTimeMS)  "RefLatencyMs"
  ms2samples/1(Samples) -> TOP/1
  Captured Tune Const/1 -> ms2samples/2(MaxLatencySamples)

== system Model_TranslationEngine64/ModelPreAmp/DecRate/AudioPilot35/Audiopilot_3_5/NoiseEstimationVariant/RegularNoiseEstimation/LFNoiseEstimatorCoh/LfNoiseImpulseRejection/Gamma0 ==
  TOP : TOP/TOP  TriggerInit=[475 20 675 70]  TopName=Gamma0  DataTypeOut=single  BankNumber=0  PreOverlay=false  PostOverlay=false  Role=Automatic
      settings: SourceProductName=Bose Talaria
  TimeConstant2Coefficient : MATLAB Function  TreatAsAtomicUnit=on
  TranslateTrigger : TuneVar/TranslateTrigger  TriggerInit=[306 -100 344 -45]
      settings: SourceProductName=Bose Talaria
  Tune Variable : TuneVar/TuneVar  TuneName=Gamma0TauS  SpecifyMaxSize=off  VariableDim=1 (Row)  MaxSize=[1 1]  TunabilityNumber=1  MinValue=[]  MaxValue=[]  TriggerInit=[-160 22 155 68]  MaskValue=Config.ImpRejGamma0TauSec
      settings: SourceProductName=Bose Talaria
  wires:
  Tune Variable/1 -> TimeConstant2Coefficient/1(tau)  "Gamma0TauS"
  TimeConstant2Coefficient/1(coef) -> TOP/1
  TranslateTrigger/1 -> TimeConstant2Coefficient/Trigger

== system Model_TranslationEngine64/ModelPreAmp/DecRate/AudioPilot35/Audiopilot_3_5/NoiseEstimationVariant/RegularNoiseEstimation/LFNoiseEstimatorCoh/LfNoiseImpulseRejection/ImpulseVarianceFilterCoef ==
  TOP : TOP/TOP  TriggerInit=[440 17 725 83]  TopName=ImpulseVarianceFilterCoef  DataTypeOut=single  BankNumber=0  PreOverlay=false  PostOverlay=false  Role=Automatic
      settings: SourceProductName=Bose Talaria
  TimeConstant2Coefficient : MATLAB Function  TreatAsAtomicUnit=on
  TranslateTrigger : TuneVar/TranslateTrigger  TriggerInit=[306 -100 344 -45]
      settings: SourceProductName=Bose Talaria
  Tune Variable : TuneVar/TuneVar  TuneName=ImpulseVarianceFiltTauS  SpecifyMaxSize=off  VariableDim=1 (Row)  MaxSize=[1 1]  TunabilityNumber=1  MinValue=[]  MaxValue=[]  TriggerInit=[-265 20 100 80]  MaskValue=Config.ImpRejImpulseVarianceFilterTauSec
      settings: SourceProductName=Bose Talaria
  wires:
  Tune Variable/1 -> TimeConstant2Coefficient/1(tau)  "ImpulseVarianceFiltTauS"
  TimeConstant2Coefficient/1(coef) -> TOP/1
  TranslateTrigger/1 -> TimeConstant2Coefficient/Trigger

== system Model_TranslationEngine64/ModelPreAmp/DecRate/AudioPilot35/Audiopilot_3_5/NoiseEstimationVariant/RegularNoiseEstimation/LFNoiseEstimatorCoh/LfNoiseImpulseRejection/ImpulseVarianceScale ==
  TOP : TOP/TOP  TriggerInit=[440 20 585 80]  TopName=ImpulseVarianceScale  DataTypeOut=single  BankNumber=BankNumber  PreOverlay=PreOverlay  PostOverlay=PostOverlay  Role=Automatic
      settings: SourceProductName=Bose Talaria
  TrivialTranslation : TuneVar/TrivialTranslation  TriggerInit=[300 28 350 72]
      settings: SourceProductName=Bose Talaria
  Tune Variable : TuneVar/TuneVar  TuneName=ImpulseVarianceScale  SpecifyMaxSize=off  VariableDim=1 (Row)  MaxSize=[1 1]  TunabilityNumber=1  MinValue=MinValue  MaxValue=MaxValue  TriggerInit=[20 25 190 75]  MaskValue=MaskValue
      settings: SourceProductName=Bose Talaria
  wires:
  TrivialTranslation/1 -> TOP/1
  Tune Variable/1 -> TrivialTranslation/1  "ImpulseVarianceScale"

== system Model_TranslationEngine64/ModelPreAmp/DecRate/AudioPilot35/Audiopilot_3_5/NoiseEstimationVariant/RegularNoiseEstimation/LFNoiseEstimatorCoh/LfNoiseImpulseRejection/MusicVarianceScale ==
  TOP : TOP/TOP  TriggerInit=[440 20 585 80]  TopName=MusicVarianceScale  DataTypeOut=single  BankNumber=BankNumber  PreOverlay=PreOverlay  PostOverlay=PostOverlay  Role=Automatic
      settings: SourceProductName=Bose Talaria
  TrivialTranslation : TuneVar/TrivialTranslation  TriggerInit=[300 28 350 72]
      settings: SourceProductName=Bose Talaria
  Tune Variable : TuneVar/TuneVar  TuneName=MusicVarianceScale  SpecifyMaxSize=off  VariableDim=1 (Row)  MaxSize=[1 1]  TunabilityNumber=1  MinValue=MinValue  MaxValue=MaxValue  TriggerInit=[20 25 190 75]  MaskValue=MaskValue
      settings: SourceProductName=Bose Talaria
  wires:
  TrivialTranslation/1 -> TOP/1
  Tune Variable/1 -> TrivialTranslation/1  "MusicVarianceScale"

== system Model_TranslationEngine64/ModelPreAmp/DecRate/AudioPilot35/Audiopilot_3_5/NoiseEstimationVariant/RegularNoiseEstimation/LFNoiseEstimatorCoh/LfNoiseImpulseRejection/NoiseVarianceScale ==
  TOP : TOP/TOP  TriggerInit=[440 20 585 80]  TopName=NoiseVarianceScale  DataTypeOut=single  BankNumber=BankNumber  PreOverlay=PreOverlay  PostOverlay=PostOverlay  Role=Automatic
      settings: SourceProductName=Bose Talaria
  TrivialTranslation : TuneVar/TrivialTranslation  TriggerInit=[300 28 350 72]
      settings: SourceProductName=Bose Talaria
  Tune Variable : TuneVar/TuneVar  TuneName=NoiseVarianceScale  SpecifyMaxSize=off  VariableDim=1 (Row)  MaxSize=[1 1]  TunabilityNumber=1  MinValue=MinValue  MaxValue=MaxValue  TriggerInit=[20 25 190 75]  MaskValue=MaskValue
      settings: SourceProductName=Bose Talaria
  wires:
  TrivialTranslation/1 -> TOP/1
  Tune Variable/1 -> TrivialTranslation/1  "NoiseVarianceScale"

== system Model_TranslationEngine64/ModelPreAmp/DecRate/AudioPilot35/Audiopilot_3_5/NoiseEstimationVariant/RegularNoiseEstimation/LFNoiseEstimatorCoh/LfNoiseImpulseRejection/OutputMin  ==
  TOP : TOP/TOP  TriggerInit=[440 20 585 80]  TopName=OutputMin  DataTypeOut=single  BankNumber=BankNumber  PreOverlay=PreOverlay  PostOverlay=PostOverlay  Role=Automatic
      settings: SourceProductName=Bose Talaria
  TrivialTranslation : TuneVar/TrivialTranslation  TriggerInit=[300 28 350 72]
      settings: SourceProductName=Bose Talaria
  Tune Variable : TuneVar/TuneVar  TuneName=OutputMin  SpecifyMaxSize=off  VariableDim=1 (Row)  MaxSize=[1 1]  TunabilityNumber=1  MinValue=MinValue  MaxValue=MaxValue  TriggerInit=[20 25 190 75]  MaskValue=MaskValue
      settings: SourceProductName=Bose Talaria
  wires:
  TrivialTranslation/1 -> TOP/1
  Tune Variable/1 -> TrivialTranslation/1  "OutputMin"

== system Model_TranslationEngine64/ModelPreAmp/DecRate/AudioPilot35/Audiopilot_3_5/NoiseEstimationVariant/RegularNoiseEstimation/LFNoiseEstimatorCoh/LfPreProcess/FilterMic ==
  InnerLink : Subsystem  mask(Bose Pool IIR Tunable){FeatureName=Mic, Config=InnerLinkConfig}
      mask prompts: FeatureName "Filter name/purpose"; Config "PoolIirTunableConfig"
      mask help:
      | Pool IIR Tunable is a configurable multi-channel IIR filter that supports one or more channels. This block offers flexibility of tuning the number of stages and coefficients. Different filter coefficients and number of stages (biquads) can be used for each channel filter. The Pool IIR Tunable block supports different implementations, which could be configured at build-time:
      |
      | (i)   Generic: IIR filter code not optimized for any processor
      | (ii)  SharcCore: IIR filters executing on core (uses pooliir.asm CRL)
      | (iii) SharcGulAccel: IIR filters executing on IIR hardware accelerator, offloading MIPS usage from core
      | (iv) SharcGxpAccel: IIR filters take advantage of additional accelerators available on GXP processor
      | (v)  Hexagon: TBD
      |
      | NOTE: When using Pool IIR for Sharc-plus based processors, the codeWorkMemory buffer and input buffer should always be mapped to L1 memory to optimize MIPS utilization and avoid audio artifacts.
      |
      | For more information, please see 'Help'.
      mask init:
      | blkh=gcbh;
      | Config=BTConfig.Assert(blkh,Config);
      | 
      | Config.Validate();
      | Config.DoMaskInit(blkh);
      mask Help:
      | <b>Input signals: </b>
      | AudioIn: input channels [frame size x number of channels]
      | 
      | <b>Output signals: </b>
      | AudioOut: output channels [frame size x number of channels]
      | 
      | <b>Mask parameters: </b>
      | PoolIirTunableConfig
      | Filter name/purpose
      mask TypeOptions FeatureName: PoolIirTunableWithReset/FeatureName
      mask Display: DrawPoolIirIcon;

== system Model_TranslationEngine64/ModelPreAmp/DecRate/AudioPilot35/Audiopilot_3_5/NoiseEstimationVariant/RegularNoiseEstimation/LFNoiseEstimatorCoh/LfPreProcess/FilterRef ==
  InnerLink : Subsystem  mask(Bose Pool IIR Tunable){FeatureName=Ref, Config=InnerLinkConfig}
      mask prompts: FeatureName "Filter name/purpose"; Config "PoolIirTunableConfig"
      mask help:
      | Pool IIR Tunable is a configurable multi-channel IIR filter that supports one or more channels. This block offers flexibility of tuning the number of stages and coefficients. Different filter coefficients and number of stages (biquads) can be used for each channel filter. The Pool IIR Tunable block supports different implementations, which could be configured at build-time:
      |
      | (i)   Generic: IIR filter code not optimized for any processor
      | (ii)  SharcCore: IIR filters executing on core (uses pooliir.asm CRL)
      | (iii) SharcGulAccel: IIR filters executing on IIR hardware accelerator, offloading MIPS usage from core
      | (iv) SharcGxpAccel: IIR filters take advantage of additional accelerators available on GXP processor
      | (v)  Hexagon: TBD
      |
      | NOTE: When using Pool IIR for Sharc-plus based processors, the codeWorkMemory buffer and input buffer should always be mapped to L1 memory to optimize MIPS utilization and avoid audio artifacts.
      |
      | For more information, please see 'Help'.
      mask init:
      | blkh=gcbh;
      | Config=BTConfig.Assert(blkh,Config);
      | 
      | Config.Validate();
      | Config.DoMaskInit(blkh);
      mask Help:
      | <b>Input signals: </b>
      | AudioIn: input channels [frame size x number of channels]
      | 
      | <b>Output signals: </b>
      | AudioOut: output channels [frame size x number of channels]
      | 
      | <b>Mask parameters: </b>
      | PoolIirTunableConfig
      | Filter name/purpose
      mask TypeOptions FeatureName: PoolIirTunableWithReset/FeatureName
      mask Display: DrawPoolIirIcon;

== system Model_TranslationEngine64/ModelPreAmp/DecRate/AudioPilot35/Audiopilot_3_5/NoiseEstimationVariant/RegularNoiseEstimation/LFNoiseEstimatorCoh/ReferenceLatency/RefLatencySamples ==
  Captured Tune Const : CapturedConstLib/CapturedConst  TriggerInit=[70 162 170 198]  Role=Automatic
      settings: SourceProductName=Bose Talaria
  TOP : TOP/TOP  TriggerInit=[410 120 555 180]  TopName=RefLatencySamples  DataTypeOut=int32  BankNumber=0  PreOverlay=false  PostOverlay=false  Role=Automatic
      settings: SourceProductName=Bose Talaria
  TranslateTrigger : TuneVar/TranslateTrigger  TriggerInit=[286 -35 324 20]
      settings: SourceProductName=Bose Talaria
  Tune Variable : TuneVar/TuneVar  TuneName=RefLatencyMs  SpecifyMaxSize=off  VariableDim=1 (Row)  MaxSize=[1 1]  TunabilityNumber=1  MinValue=[]  MaxValue=[]  TriggerInit=[-245 90 -55 140]  MaskValue=Config.RefLatencyMsec
      settings: SourceProductName=Bose Talaria
  ms2samples : MATLAB Function  TreatAsAtomicUnit=on
  wires:
  Tune Variable/1 -> ms2samples/1(DelayTimeMS)  "RefLatencyMs"
  ms2samples/1(Samples) -> TOP/1
  TranslateTrigger/1 -> ms2samples/Trigger
  Captured Tune Const/1 -> ms2samples/2(MaxLatencySamples)
